simulink model "untitled"  (R2021a)
settings: Solver=VariableStepAuto  StartTime=0.0  StopTime=900  RelTol=1e-3
settings Model: Creator=Nestor  LastModifiedBy=Nestor

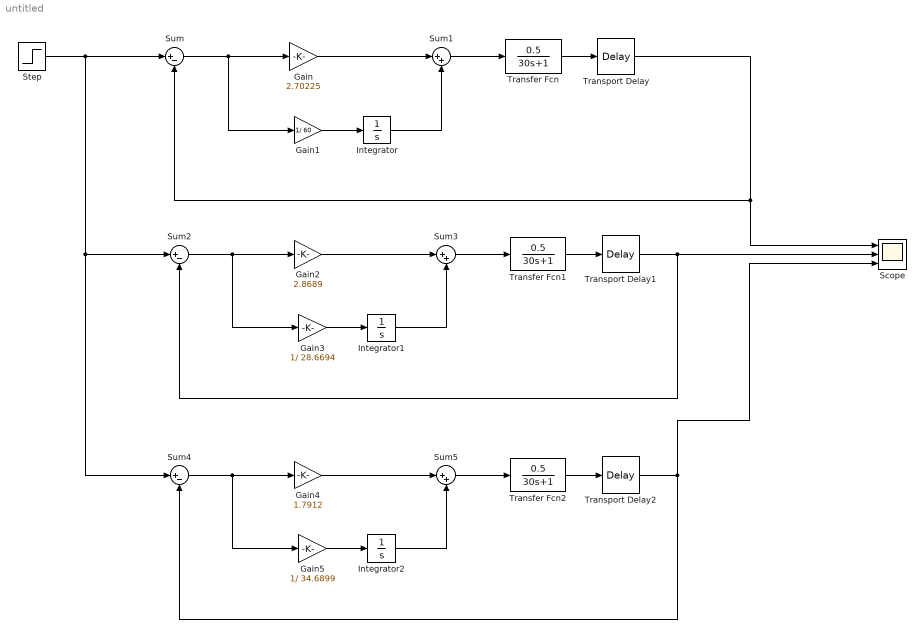
== system untitled ==
  Gain : Gain  Gain=2.70225
  Gain1 : Gain  Gain=1/ 60
  Gain2 : Gain  Gain=2.8689
  Gain3 : Gain  Gain=1/ 28.6694
  Gain4 : Gain  Gain=1.7912
  Gain5 : Gain  Gain=1/ 34.6899
  Integrator : Integrator
  Integrator1 : Integrator
  Integrator2 : Integrator
  Scope : Scope  NumInputPorts=3
  Step : Step  SampleTime=0
  Sum : Sum  Inputs=|+-
  Sum1 : Sum  Inputs=|++
  Sum2 : Sum  Inputs=|+-
  Sum3 : Sum  Inputs=|++
  Sum4 : Sum  Inputs=|+-
  Sum5 : Sum  Inputs=|++
  Transfer Fcn : TransferFcn  Numerator=[0.5]  Denominator=[30 1]
  Transfer Fcn1 : TransferFcn  Numerator=[0.5]  Denominator=[30 1]
  Transfer Fcn2 : TransferFcn  Numerator=[0.5]  Denominator=[30 1]
  Transport Delay : TransportDelay  DelayTime=20
  Transport Delay1 : TransportDelay  DelayTime=20
  Transport Delay2 : TransportDelay  DelayTime=20
  wires:
  Transfer Fcn/1 -> Transport Delay/1
  Sum/1 -> Gain1/1, Gain/1
  Gain/1 -> Sum1/1
  Sum1/1 -> Transfer Fcn/1
  Transport Delay/1 -> Sum/2, Scope/1
  Gain1/1 -> Integrator/1
  Integrator/1 -> Sum1/2
  Sum2/1 -> Gain3/1, Gain2/1
  Gain2/1 -> Sum3/1
  Sum3/1 -> Transfer Fcn1/1
  Transfer Fcn1/1 -> Transport Delay1/1
  Transport Delay1/1 -> Scope/2, Sum2/2
  Gain3/1 -> Integrator1/1
  Integrator1/1 -> Sum3/2
  Sum4/1 -> Gain5/1, Gain4/1
  Gain4/1 -> Sum5/1
  Sum5/1 -> Transfer Fcn2/1
  Transfer Fcn2/1 -> Transport Delay2/1
  Step/1 -> Sum4/1, Sum2/1, Sum/1
  Transport Delay2/1 -> Scope/3, Sum4/2
  Gain5/1 -> Integrator2/1
  Integrator2/1 -> Sum5/2
